simulink model "active_cell_4s"  (R2020a)
settings: Solver=VariableStepAuto  StartTime=0.0  StopTime=15  RelTol=1e-3
undefined symbols (not defined in the file or in its folder): Ion, Lithium
libraries: powerlib x25, electricdrivelib x4, powerlib_meascontrol x1
settings Model: Creator=LEGION  LastModifiedBy=LEGION

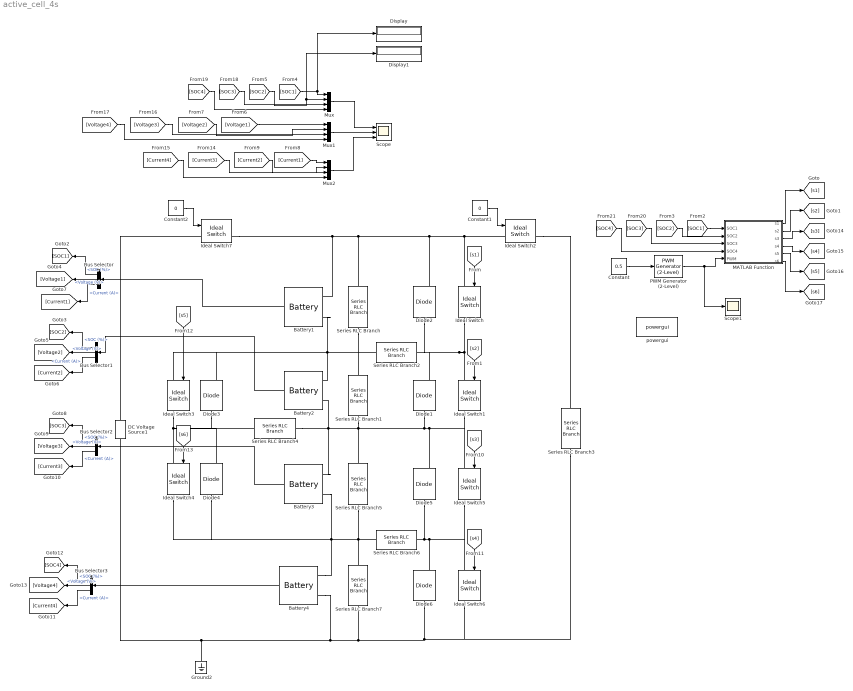
== system active_cell_4s ==
  Battery1 : electricdrivelib/Extra Sources/Battery  BatType=Lithium-Ion  ShowTempParam=off  ThermalPreset=no  ShowAgeParam=off  NomV=3.7  NomQ=3  SOC=50  Batt_Tr=30  PresetModel=on  MaxQ=3  MinV=2.775  FullV=4.3068  Dis_rate=1.3043  R=0.012333  Normal_OP=2.713  expZone="[3.9974     0.14739]"  current=[6.5 13 32.5]  Units=Time  Tci=20  NomT=20  T2=-30  MaxQ2=4.8  FullV2=7.1  Normal_OP2=5.655  expZone2="[6.58           1]"  Rca=0.6  ti=2000  Dp=0  Neq0=0  Tsim=1e6  Ta1=25  Qeol=5.4*0.9  Reol=0.013333*1.2  Char_age=[2.3478, 3]  Dis_age=[2.3478, 10]  N1=1500  N2=10500  N3=1000  N4=1400  Ta2=45  N5=950
  Battery2 : electricdrivelib/Extra Sources/Battery  BatType=Lithium-Ion  ShowTempParam=off  ThermalPreset=no  ShowAgeParam=off  NomV=3.7  NomQ=3  SOC=40  Batt_Tr=30  PresetModel=on  MaxQ=3  MinV=2.775  FullV=4.3068  Dis_rate=1.3043  R=0.012333  Normal_OP=2.713  expZone="[3.9974     0.14739]"  current=[6.5 13 32.5]  Units=Time  Tci=20  NomT=20  T2=-30  MaxQ2=4.8  FullV2=7.1  Normal_OP2=5.655  expZone2="[6.58           1]"  Rca=0.6  ti=2000  Dp=0  Neq0=0  Tsim=1e6  Ta1=25  Qeol=5.4*0.9  Reol=0.013333*1.2  Char_age=[2.3478, 3]  Dis_age=[2.3478, 10]  N1=1500  N2=10500  N3=1000  N4=1400  Ta2=45  N5=950
  Battery3 : electricdrivelib/Extra Sources/Battery  BatType=Lithium-Ion  ShowTempParam=off  ThermalPreset=no  ShowAgeParam=off  NomV=3.7  NomQ=3  SOC=30  Batt_Tr=30  PresetModel=on  MaxQ=3  MinV=2.775  FullV=4.3068  Dis_rate=1.3043  R=0.012333  Normal_OP=2.713  expZone="[3.9974     0.14739]"  current=[6.5 13 32.5]  Units=Time  Tci=20  NomT=20  T2=-30  MaxQ2=4.8  FullV2=7.1  Normal_OP2=5.655  expZone2="[6.58           1]"  Rca=0.6  ti=2000  Dp=0  Neq0=0  Tsim=1e6  Ta1=25  Qeol=5.4*0.9  Reol=0.013333*1.2  Char_age=[2.3478, 3]  Dis_age=[2.3478, 10]  N1=1500  N2=10500  N3=1000  N4=1400  Ta2=45  N5=950
  Battery4 : electricdrivelib/Extra Sources/Battery  BatType=Lithium-Ion  ShowTempParam=off  ThermalPreset=no  ShowAgeParam=off  NomV=3.7  NomQ=3  SOC=20  Batt_Tr=30  PresetModel=on  MaxQ=3  MinV=2.775  FullV=4.3068  Dis_rate=1.3043  R=0.012333  Normal_OP=2.713  expZone="[3.9974     0.14739]"  current=[6.5 13 32.5]  Units=Time  Tci=20  NomT=20  T2=-30  MaxQ2=4.8  FullV2=7.1  Normal_OP2=5.655  expZone2="[6.58           1]"  Rca=0.6  ti=2000  Dp=0  Neq0=0  Tsim=1e6  Ta1=25  Qeol=5.4*0.9  Reol=0.013333*1.2  Char_age=[2.3478, 3]  Dis_age=[2.3478, 10]  N1=1500  N2=10500  N3=1000  N4=1400  Ta2=45  N5=950
  Bus Selector{,1..3} (4 alike) : BusSelector  OutputSignals=SOC (%),Voltage (V),Current (A)
  Constant : Constant  Value=0.5
  Constant1 : Constant  Value=0
  Constant2 : Constant  Value=0
  DC Voltage Source1 : powerlib/Electrical Sources/DC Voltage Source  Amplitude=12  Measurements=None
  Diode{1..6} (6 alike) : powerlib/Power Electronics/Diode  Ron=0.001  Lon=0  Vf=0.8  IC=0  UseSnubber=0  Rs=500  Cs=250e-9  Measurements=on
  Display : Display
  Display1 : Display
  Ground2 : powerlib/Elements/Ground  LConnTagsString=a
  Ideal Switch{,1..7} (8 alike) : powerlib/Power Electronics/Ideal Switch  Ron=0.001  Lon=0  IC=0  Rs=1e5  Cs=inf  Measurements=on
  MATLAB Function : MATLAB Function  TreatAsAtomicUnit=on
  Mux : Mux
  Mux1 : Mux
  Mux2 : Mux
  PWM Generator (2-Level) : powerlib_meascontrol/Pulse & Signal Generators/PWM Generator (2-Level)  ModulatorType=Single-phase half-bridge (2 pulses)  ModulatorMode=Unsynchronized  Fc=500  Pc=0  nF=27  MinMax="[ -1  1 ]"  SamplingTechnique=Natural  ModulatingSignals=off  m=0.8  Freq=60  Phase=0  Ts=0  ShowCarrierOutport=off
  Scope : Scope  NumInputPorts=3
  Scope1 : Scope
  Series RLC Branch{,1,5,7} (4 alike) : powerlib/Elements/Series RLC Branch  LConnTagsString=__new0  RConnTagsString=__new0  BranchType=C  Resistance=1  Inductance=1e-3  SetiL0=off  InitialCurrent=0  Capacitance=1e-6  Setx0=off  InitialVoltage=0  Measurements=None
  Series RLC Branch2 : powerlib/Elements/Series RLC Branch  LConnTagsString=__new0  RConnTagsString=__new0  BranchType=L  Resistance=1  Inductance=1e-3  SetiL0=off  InitialCurrent=0  Capacitance=1e-6  Setx0=off  InitialVoltage=0  Measurements=None
  Series RLC Branch3 : powerlib/Elements/Series RLC Branch  LConnTagsString=__new0  RConnTagsString=__new0  BranchType=R  Resistance=1  Inductance=1e-3  SetiL0=off  InitialCurrent=0  Capacitance=1e-6  Setx0=off  InitialVoltage=0  Measurements=None
  Series RLC Branch4 : powerlib/Elements/Series RLC Branch  LConnTagsString=__new0  RConnTagsString=__new0  BranchType=L  Resistance=1  Inductance=1e-3  SetiL0=off  InitialCurrent=0  Capacitance=1e-6  Setx0=off  InitialVoltage=0  Measurements=None
  Series RLC Branch6 : powerlib/Elements/Series RLC Branch  LConnTagsString=__new0  RConnTagsString=__new0  BranchType=L  Resistance=1  Inductance=1e-3  SetiL0=off  InitialCurrent=0  Capacitance=1e-6  Setx0=off  InitialVoltage=0  Measurements=None
  powergui : powerlib/powergui  Priority=1  SimulationMode=Discrete  SampleTime=50e-5  frequency=60  Iterations=50  frequencyindice=0  Pbase=100e6  ErrMax=1e-4  UnitsV=kV  UnitsW=MW  buscounter=0  FunctionMessages=off  echomessages=off  EnableUseOfTLC=off  CurrentSourceSwitches=off  DisableSnubberDevices=off  DisableRonSwitches=off  DisableVfSwitches=off  DisplayEquations=off  AutomaticDiscreteSolvers=off  SolverType=Tustin/Backward Euler (TBE)  Interpol=off  ExternalGateDelay=off  methode=off  Ts=100  x0status=blocks  SPID=on  SwTol=0  HookPort=off  NonlinearTolerance=1e-4  nMaxIteration=100  ContinueOnMaxIteration=off  RestoreLinks=warning  ResistiveCurrentMeasurement=off  Frange=[0:2:500]  Ylog=off  Xlog=on  ShowGrid=off  save=off  variable=ZData  structure=0  ZoomFFT=off  StartTime=0.0  cycles=1  DisplayStyle=1  fundamental=60  FreqAxis=off  MaxFrequency=1000  frequencyindicesteady=1  RmsSteady=1  display=off
  wires:
  [s1] -> Ideal Switch/1
  [s2] -> Ideal Switch1/1
  Battery1/1 -> Bus Selector/1
  Battery2/1 -> Bus Selector1/1
  Bus Selector/1 -> [SOC1]  "<SOC (%)>"
  Bus Selector1/1 -> [SOC2]  "<SOC (%)>"
  MATLAB Function/1(s1) -> [s1]
  MATLAB Function/2(s2) -> [s2]
  Bus Selector/2 -> [Voltage1]  "<Voltage (V)>"
  Bus Selector1/2 -> [Voltage2]  "<Voltage (V)>"
  Bus Selector/3 -> [Current1]  "<Current (A)>"
  Bus Selector1/3 -> [Current2]  "<Current (A)>"
  Mux/1 -> Scope/1
  [SOC1] -> Display/1, Mux/1
  [SOC2] -> Display1/1, Mux/2
  Mux1/1 -> Scope/2
  [Voltage1] -> Mux1/1
  [Voltage2] -> Mux1/2
  [Current1] -> Mux2/1
  [Current2] -> Mux2/2
  Mux2/1 -> Scope/3
  Constant1/1 -> Ideal Switch2/1
  Constant/1 -> PWM Generator (2-Level)/1
  PWM Generator (2-Level)/1 -> Scope1/1, MATLAB Function/5(PWM)
  [SOC2] -> MATLAB Function/2(SOC2)
  [SOC1] -> MATLAB Function/1(SOC1)
  Constant2/1 -> Ideal Switch7/1
  Bus Selector2/3 -> [Current3]  "<Current (A)>"
  Bus Selector2/2 -> [Voltage3]  "<Voltage (V)>"
  Battery3/1 -> Bus Selector2/1
  Bus Selector2/1 -> [SOC3]  "<SOC (%)>"
  Battery4/1 -> Bus Selector3/1
  Bus Selector3/2 -> [Voltage4]  "<Voltage (V)>"
  Bus Selector3/3 -> [Current4]  "<Current (A)>"
  Bus Selector3/1 -> [SOC4]  "<SOC (%)>"
  [s3] -> Ideal Switch5/1
  [s4] -> Ideal Switch6/1
  [s5] -> Ideal Switch3/1
  [s6] -> Ideal Switch4/1
  [Current3] -> Mux2/3
  [Current4] -> Mux2/4
  [Voltage3] -> Mux1/3
  [Voltage4] -> Mux1/4
  [SOC3] -> Mux/3
  [SOC4] -> Mux/4
  [SOC3] -> MATLAB Function/3(SOC3)
  [SOC4] -> MATLAB Function/4(SOC4)
  MATLAB Function/3(s3) -> [s3]
  MATLAB Function/4(s4) -> [s4]
  MATLAB Function/5(s5) -> [s5]
  MATLAB Function/6(s6) -> [s6]
  connections:
  Ideal Switch/LConn1 -- Ideal Switch2/LConn1 -- Diode2/RConn1 -- Ideal Switch7/RConn1 -- Battery1/LConn1 -- Series RLC Branch/LConn1
  Ideal Switch/RConn1 -- Diode2/LConn1 -- Series RLC Branch2/RConn1 -- Diode1/RConn1 -- Ideal Switch1/LConn1
  Diode1/LConn1 -- Ideal Switch1/RConn1 -- Ideal Switch5/LConn1 -- Diode5/RConn1 -- Series RLC Branch1/RConn1 -- Series RLC Branch5/LConn1 -- Battery2/LConn2 -- Battery3/LConn1 -- Series RLC Branch4/RConn1
  Battery1/LConn2 -- Diode3/RConn1 -- Ideal Switch3/LConn1 -- Series RLC Branch1/LConn1 -- Series RLC Branch2/LConn1 -- Series RLC Branch/RConn1 -- Battery2/LConn1
  Ideal Switch2/RConn1 -- Series RLC Branch3/LConn1
  Ideal Switch3/RConn1 -- Series RLC Branch4/LConn1 -- Diode4/RConn1 -- Diode3/LConn1 -- Ideal Switch4/LConn1
  Series RLC Branch5/RConn1 -- Series RLC Branch7/LConn1 -- Ideal Switch4/RConn1 -- Diode4/LConn1 -- Battery3/LConn2 -- Battery4/LConn1 -- Series RLC Branch6/LConn1
  Diode5/LConn1 -- Ideal Switch6/LConn1 -- Ideal Switch5/RConn1 -- Diode6/RConn1 -- Series RLC Branch6/RConn1
  Ground2/LConn1 -- DC Voltage Source1/LConn1 -- Battery4/LConn2 -- Series RLC Branch3/RConn1 -- Ideal Switch6/RConn1 -- Diode6/LConn1 -- Series RLC Branch7/RConn1
  Ideal Switch7/LConn1 -- DC Voltage Source1/RConn1

== matlab function active_cell_4s/MATLAB Function ==
  data: SOC1 input; s1 output; SOC2 input; SOC3 input; SOC4 input; PWM input; s2 output; s3 output; s4 output; s5 output; s6 output
function [s1,s2,s3,s4,s5,s6] = fcn(SOC1, SOC2, SOC3, SOC4, PWM)
%#codegen
SOC1 = SOC1(1);
SOC2 = SOC2(1);
SOC3 = SOC3(1);
SOC4 = SOC4(1);
PWM = PWM(1);
% Inisialisasi output
s1 = 0;
s2 = 0;
if SOC2<SOC1
    s1=PWM;
    s2=0;
elseif SOC1<SOC2
    s1=0;
    s2=PWM;
else 
    s1=0;
    s2=0;      
end
